simulink model "MODELSIMTOANHETHONG"  (R2020a)
settings: Solver=VariableStepAuto  StartTime=0.0  StopTime=2  RelTol=1e-3
InitFcn:
  | Kp1=65;
  | Ki1=10;
  | Kp2=65;
  | Ki2=45;
  | Kp3=60;
  | Ki3=30;
  | Kp4=60;
  | Ki4=25;
  | Phir=0.2;
undefined symbols (not defined in the file): DiscIntNeverNeededParam, sigbuilder_block
libraries: powerlib x11, modelsimlib x8
settings Model: Creator=Admin  LastModifiedBy=Admin
settings SolverCC: ZeroCrossAlgorithm=Adaptive
settings DebuggingCC: IgnoredZcDiagnostic=none  UnconnectedInputMsg=none  UnconnectedOutputMsg=none  UnconnectedLineMsg=none
settings ModelReferenceCC: EnableRefExpFcnMdlSchedulingChecks=off
settings RTWCC: Description=Generic Real-Time Target

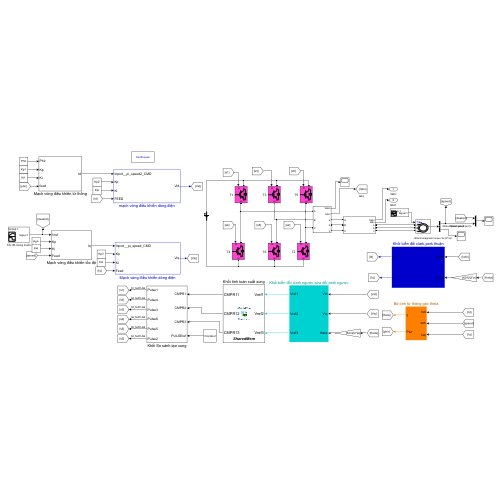
[thumbnail: Simulink's stored preview of the top-level diagram]
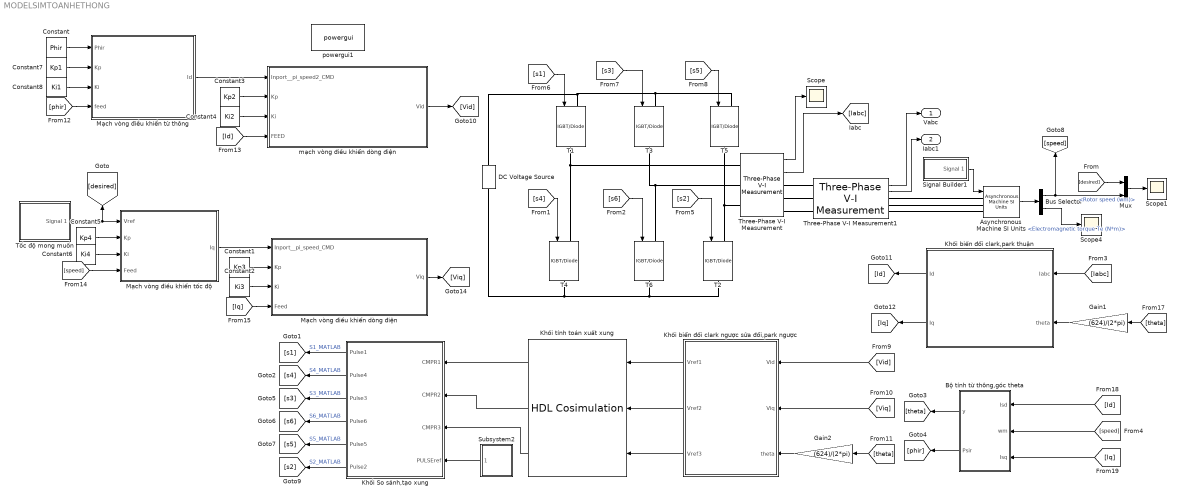
== system MODELSIMTOANHETHONG ==
  Asynchronous Machine SI Units : powerlib/Machines/Asynchronous Machine SI Units  RotorType=Squirrel-cage  PresetModel=No  MechanicalLoad=Torque Tm  ShowDetailedParameters=on  ReferenceFrame=Rotor  Units=SI  MeasurementBus=off  NominalParameters=[40000 380 50]  VoltageRatio=1  Stator=[1.912 0.005974]  Rotor=[1.112 0.005974]  Cage1=[ 0.022 0.226/377]  Cage2=[ 0.022 0.226/377]  Lm=0.2358  Mechanical=[0.4 0 2]  PolePairs=2  InitialConditions=[1 0 0 0 0 0 0 0]  SimulateSaturation=off  Saturation=[14.03593122, 27.81365428, 53.79336849, 72.68890987, 97.98006896, 148.6815601, 215.7428561, 302.9841135, 420.4778367 ; 230, 322, 414, 460, 506, 552, 598, 644, 690]  LoadFlowParameters=1492000  TsPowergui=0  TsBlock=-1  IterativeModel=Trapezoidal non iterative  IterativeDiscreteModel=Trapezoidal non iterative  Pmec=1.492e+006
  Bus Selector : BusSelector  OutputSignals=Mechanical.Rotor speed (wm),Mechanical.Electromagnetic torque Te (N*m)
  Bộ tính từ thông,góc theta : Subsystem
  Constant : Constant  Value=Phir
  Constant1 : Constant  Value=Kp3
  Constant2 : Constant  Value=Ki3
  Constant3 : Constant  Value=Kp2
  Constant4 : Constant  Value=Ki2
  Constant5 : Constant  Value=Kp4
  Constant6 : Constant  Value=Ki4
  Constant7 : Constant  Value=Kp1
  Constant8 : Constant  Value=Ki1
  DC Voltage Source : powerlib/Electrical Sources/DC Voltage Source  Amplitude=515  Measurements=None
  Gain1 : Gain  Gain=(624)/(2*pi)
  Gain2 : Gain  Gain=(624)/(2*pi)
  Khối So sánh,tạo xung : Subsystem
  Khối biến đổi clark,park thuận : Subsystem
  Khối biển đổi clark ngược sửa đổi,park ngược : Subsystem
  Khối tính toán xuất xung : modelsimlib/HDL Cosimulation  PortPaths=/cmpr/Vref1;/cmpr/Vref2;/cmpr/Vref3;/cmpr/CMPR11;/cmpr/CMPR12;/cmpr/CMPR13  PortModes=[1 1 1 2 2 2 ]  PortTimes=[-1,-1,-1,2e-7,2e-7,2e-7]  PortSigns=[-1 -1 -1 -1 -1 -1 ]  PortFracLengths=[0,0,0,0,0,0]  PortWordLengths=[-1,-1,-1,24,24,24]  PortHDLWordSizes=[12,12,12,24,24,24]  CommLocal=on  CommSharedMemory=on  CommPortNumber=4449  CommShowInfo=on  ClockPaths=/cmpr/clk;/cmpr/clk200n  ClockModes=[2 2 ]  ClockTimes=[100e-9,100e-9]  TclPreSimCommand="puts \"Running Simulink Cosimulation block.\""  TclPostSimCommand="puts \"done\""  TimingMode=s  TimingScaleFactor=1  idxCellArray={'UNUSED_VAR'}  CosimBypass=Full Simulation  AllowDirectFeedthrough=on  ProductName=EDA Simulator Link MQ  RunAutoTimescale=off  HdlClocks=0  PreRunTime=0  PreRunTimeUnit=ns
  Mux : Mux  Inputs=2
  Mạch vòng điều khiển dòng điện : Subsystem
  Mạch vòng điều khiển tốc độ : Subsystem
  Mạch vòng điều khiển từ thông : Subsystem
  Scope : Scope
  Scope1 : Scope
  Scope4 : Scope
  Signal Builder1 : Subsystem  Tag=STV Subsys  LoadFcn=sigbuilder_block('load');  StartFcn=sigbuilder_block('start');  StopFcn=sigbuilder_block('stop');  ClipboardFcn=sigbuilder_block('clipboard');  mask(Sigbuilder block){tuvar=[0:10]}
      mask help: Simulink:masks:SigbuilderBlock_MD
      mask init:
      | if ~strcmp(get_param(bdroot(gcbh),'SimulationStatus'),'stopped') tuvar = sigbuilder_block('maskInit'); end
      settings: CopyFcn=sigbuilder_block('copy');  DeleteFcn=sigbuilder_block('delete');  ModelCloseFcn=sigbuilder_block('modelClose');  PreSaveFcn=sigbuilder_block('preSave');  PauseFcn=sigbuilder_block('pause');  ContinueFcn=sigbuilder_block('continue');  NameChangeFcn=sigbuilder_block('namechange');  OpenFcn=sigbuilder_block('open',[437.25 153 550.5 359.25 ]);  CloseFcn=sigbuilder_block('close');
      mask Display: plot(0, 0, 100, 100,[2, 2, 32, 32, 2], [68, 8, 8, 68, 68],[32, 2], [38, 38], [32, 19, 2],[53, 60, 44], [32, 17, 17, 2],[16, 16, 31, 31]);txt = getActiveGroup(gcbh);text(2, 100, txt,'verticalAlignment', 'top');
  Subsystem2 : Subsystem
  T{1..6} (6 alike) : powerlib/Power Electronics/IGBT//Diode  Ron=1e-3  Rs=1e5  Cs=inf  Measurements=off
  Three-Phase V-I Measurement : powerlib/Measurements/Three-Phase V-I Measurement  VoltageMeasurement=phase-to-phase  SetLabelV=off  LabelV=Vabc  Vpu=off  VpuLL=off  CurrentMeasurement=yes  SetLabelI=off  LabelI=Iabc  Ipu=off  Pbase=100e6  Vbase=500e3  OutputType=Complex  PhasorSimulation=off  PSBequivalent=0
  Three-Phase V-I Measurement1 : powerlib/Measurements/Three-Phase V-I Measurement  VoltageMeasurement=phase-to-phase  SetLabelV=off  LabelV=Vabc  Vpu=off  VpuLL=off  CurrentMeasurement=yes  SetLabelI=off  LabelI=Iabc  Ipu=off  Pbase=100e6  Vbase=500e3  OutputType=Complex  PhasorSimulation=off  PSBequivalent=0
  Tốc độ mong muốn : Subsystem  Tag=STV Subsys  LoadFcn=sigbuilder_block('load');  StartFcn=sigbuilder_block('start');  StopFcn=sigbuilder_block('stop');  ClipboardFcn=sigbuilder_block('clipboard');  mask(Sigbuilder block){tuvar=[0:10]}
      mask help: Simulink:masks:SigbuilderBlock_MD
      mask init:
      | if ~strcmp(get_param(bdroot(gcbh),'SimulationStatus'),'stopped') tuvar = sigbuilder_block('maskInit'); end
      settings: CopyFcn=sigbuilder_block('copy');  DeleteFcn=sigbuilder_block('delete');  ModelCloseFcn=sigbuilder_block('modelClose');  PreSaveFcn=sigbuilder_block('preSave');  PauseFcn=sigbuilder_block('pause');  ContinueFcn=sigbuilder_block('continue');  NameChangeFcn=sigbuilder_block('namechange');  OpenFcn=sigbuilder_block('open',[437.25 153 550.5 359.25 ]);  CloseFcn=sigbuilder_block('close');
      mask Display: plot(0, 0, 100, 100,[2, 2, 32, 32, 2], [68, 8, 8, 68, 68],[32, 2], [38, 38], [32, 19, 2],[53, 60, 44], [32, 17, 17, 2],[16, 16, 31, 31]);txt = getActiveGroup(gcbh);text(2, 100, txt,'verticalAlignment', 'top');
  mạch vòng điều khiển dòng điện : Subsystem
  powergui1 : powerlib/powergui  Priority=1  SimulationMode=Continuous  SampleTime=50e-6  frequency=60  Iterations=50  frequencyindice=0  Pbase=100e6  ErrMax=1e-4  UnitsV=kV  UnitsW=MW  buscounter=0  FunctionMessages=off  echomessages=off  EnableUseOfTLC=off  CurrentSourceSwitches=off  DisableSnubberDevices=off  DisableRonSwitches=off  DisableVfSwitches=off  DisplayEquations=off  AutomaticDiscreteSolvers=off  SolverType=Tustin/Backward Euler (TBE)  Interpol=off  ExternalGateDelay=off  methode=off  Ts=100  x0status=blocks  SPID=on  SwTol=0  HookPort=off  NonlinearTolerance=1e-4  nMaxIteration=100  ContinueOnMaxIteration=off  RestoreLinks=warning  ResistiveCurrentMeasurement=off  Frange=[0:2:500]  Ylog=off  Xlog=on  ShowGrid=off  save=off  variable=ZData  structure=0  ZoomFFT=off  StartTime=0.0  cycles=1  DisplayStyle=1  fundamental=60  FreqAxis=off  MaxFrequency=1000  frequencyindicesteady=1  RmsSteady=1  display=off
  Vabc : Outport
  Iabc1 : Outport  Port=2
  wires:
  Bus Selector/1 -> [speed], Mux/2  "<Rotor speed (wm)>"
  Bus Selector/2 -> Scope4/1  "<Electromagnetic torque Te (N*m)>"
  [theta] -> Gain2/1
  Mux/1 -> Scope1/1
  Khối tính toán xuất xung/1 -> Khối So sánh,tạo xung/1(CMPR1)
  Khối tính toán xuất xung/2 -> Khối So sánh,tạo xung/2(CMPR2)
  Khối tính toán xuất xung/3 -> Khối So sánh,tạo xung/3(CMPR3)
  Subsystem2/1(PULSEref) -> Khối So sánh,tạo xung/4(PULSEref)
  Khối So sánh,tạo xung/1(Pulse1) -> [s1]  "S1_MATLAB"
  Khối So sánh,tạo xung/2(Pulse4) -> [s4]  "S4_MATLAB"
  Khối So sánh,tạo xung/3(Pulse3) -> [s3]  "S3_MATLAB"
  Khối So sánh,tạo xung/4(Pulse6) -> [s6]  "S6_MATLAB"
  Khối So sánh,tạo xung/5(Pulse5) -> [s5]  "S5_MATLAB"
  Khối So sánh,tạo xung/6(Pulse2) -> [s2]  "S2_MATLAB"
  Three-Phase V-I Measurement/1 -> Scope/1
  [desired] -> Mux/1
  Three-Phase V-I Measurement1/2 -> Iabc1/1
  [s1] -> T1/1
  [s6] -> T6/1
  Three-Phase V-I Measurement1/1 -> Vabc/1
  [s4] -> T4/1
  [s5] -> T5/1
  [s2] -> T2/1
  [s3] -> T3/1
  Signal Builder1/1(Signal 1) -> Asynchronous Machine SI Units/1
  Three-Phase V-I Measurement/2 -> [Iabc]
  Asynchronous Machine SI Units/1 -> Bus Selector/1
  Tốc độ mong muốn/1(Signal 1) -> [desired], Mạch vòng điều khiển tốc độ/1(Vref)
  [Id] -> Bộ tính từ thông,góc theta/1(Isd)
  [speed] -> Bộ tính từ thông,góc theta/2(wm)
  [Iq] -> Bộ tính từ thông,góc theta/3(Isq)
  Bộ tính từ thông,góc theta/1(y) -> [theta]
  Bộ tính từ thông,góc theta/2(Psir) -> [phir]
  [Vid] -> Khối biển đổi clark ngược sửa đổi,park ngược/1(Vid)
  [Viq] -> Khối biển đổi clark ngược sửa đổi,park ngược/2(Viq)
  Gain2/1 -> Khối biển đổi clark ngược sửa đổi,park ngược/3(theta)
  Khối biển đổi clark ngược sửa đổi,park ngược/1(Vref1) -> Khối tính toán xuất xung/1
  Khối biển đổi clark ngược sửa đổi,park ngược/2(Vref2) -> Khối tính toán xuất xung/2
  Khối biển đổi clark ngược sửa đổi,park ngược/3(Vref3) -> Khối tính toán xuất xung/3
  Constant/1 -> Mạch vòng điều khiển từ thông/1(Phir)
  Constant7/1 -> Mạch vòng điều khiển từ thông/2(Kp)
  Constant8/1 -> Mạch vòng điều khiển từ thông/3(Ki)
  [phir] -> Mạch vòng điều khiển từ thông/4(feed)
  Mạch vòng điều khiển từ thông/1(Id) -> mạch vòng điều khiển dòng điện/1(Inport__pi_speed2_CMD)
  Constant3/1 -> mạch vòng điều khiển dòng điện/2(Kp)
  Constant4/1 -> mạch vòng điều khiển dòng điện/3(Ki)
  [Id] -> mạch vòng điều khiển dòng điện/4(FEED)
  mạch vòng điều khiển dòng điện/1(Vid) -> [Vid]
  Constant1/1 -> Mạch vòng điều khiển dòng điện/2(Kp)
  Constant2/1 -> Mạch vòng điều khiển dòng điện/3(Ki)
  [Iq] -> Mạch vòng điều khiển dòng điện/4(Feed)
  Mạch vòng điều khiển dòng điện/1(Viq) -> [Viq]
  Constant5/1 -> Mạch vòng điều khiển tốc độ/2(Kp)
  Constant6/1 -> Mạch vòng điều khiển tốc độ/3(Ki)
  [speed] -> Mạch vòng điều khiển tốc độ/4(Feed)
  Mạch vòng điều khiển tốc độ/1(Iq) -> Mạch vòng điều khiển dòng điện/1(Inport__pi_speed_CMD)
  [theta] -> Gain1/1
  [Iabc] -> Khối biến đổi clark,park thuận/1(Iabc)
  Gain1/1 -> Khối biến đổi clark,park thuận/2(theta)
  Khối biến đổi clark,park thuận/1(Id) -> [Id]
  Khối biến đổi clark,park thuận/2(Iq) -> [Iq]
  connections:
  T2/LConn1 -- Three-Phase V-I Measurement/LConn3 -- T5/RConn1
  T6/LConn1 -- T3/RConn1 -- Three-Phase V-I Measurement/LConn2
  T1/LConn1 -- T5/LConn1 -- T3/LConn1 -- DC Voltage Source/RConn1
  T2/RConn1 -- DC Voltage Source/LConn1 -- T4/RConn1 -- T6/RConn1
  T4/LConn1 -- Three-Phase V-I Measurement/LConn1 -- T1/RConn1
  Three-Phase V-I Measurement/RConn3 -- Three-Phase V-I Measurement1/LConn3
  Asynchronous Machine SI Units/LConn2 -- Three-Phase V-I Measurement1/RConn2
  Asynchronous Machine SI Units/LConn1 -- Three-Phase V-I Measurement1/RConn1
  Asynchronous Machine SI Units/LConn3 -- Three-Phase V-I Measurement1/RConn3
  Three-Phase V-I Measurement/RConn1 -- Three-Phase V-I Measurement1/LConn1
  Three-Phase V-I Measurement1/LConn2 -- Three-Phase V-I Measurement/RConn2

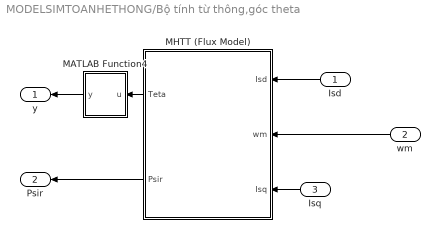
== system MODELSIMTOANHETHONG/Bộ tính từ thông,góc theta ==
  Isd : Inport
  wm : Inport  Port=2
  Isq : Inport  Port=3
  MATLAB Function4 : MATLAB Function  TreatAsAtomicUnit=on
  MHTT (Flux Model) : Subsystem
  y : Outport
  Psir : Outport  Port=2
  wires:
  wm/1 -> MHTT (Flux Model)/2(wm)
  MHTT (Flux Model)/1(Teta) -> MATLAB Function4/1(u)
  Isq/1 -> MHTT (Flux Model)/3(Isq)
  Isd/1 -> MHTT (Flux Model)/1(Isd)
  MATLAB Function4/1(y) -> y/1
  MHTT (Flux Model)/2(Psir) -> Psir/1

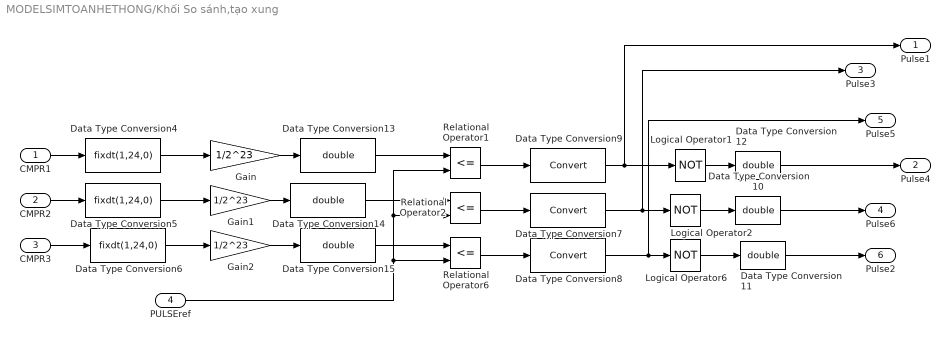
== system MODELSIMTOANHETHONG/Khối So sánh,tạo xung ==
  CMPR1 : Inport
  CMPR2 : Inport  Port=2
  CMPR3 : Inport  Port=3
  PULSEref : Inport  Port=4
  Data Type Conversion10 : DataTypeConversion  OutDataTypeStr=double
  Data Type Conversion11 : DataTypeConversion  OutDataTypeStr=double
  Data Type Conversion12 : DataTypeConversion  OutDataTypeStr=double
  Data Type Conversion13 : DataTypeConversion  OutDataTypeStr=double  SampleTime=2e-7
  Data Type Conversion14 : DataTypeConversion  OutDataTypeStr=double  SampleTime=2e-7
  Data Type Conversion15 : DataTypeConversion  OutDataTypeStr=double  SampleTime=2e-7
  Data Type Conversion4 : DataTypeConversion  OutDataTypeStr=fixdt(1,24,0)  SampleTime=2e-7
  Data Type Conversion5 : DataTypeConversion  OutDataTypeStr=fixdt(1,24,0)  SampleTime=2e-7
  Data Type Conversion6 : DataTypeConversion  OutDataTypeStr=fixdt(1,24,0)  SampleTime=2e-7
  Data Type Conversion7 : DataTypeConversion
  Data Type Conversion8 : DataTypeConversion
  Data Type Conversion9 : DataTypeConversion
  Gain : Gain  Gain=1/2^23
  Gain1 : Gain  Gain=1/2^23
  Gain2 : Gain  Gain=1/2^23
  Logical Operator1 : Logic  Operator=NOT  AllPortsSameDT=off
  Logical Operator2 : Logic  Operator=NOT  AllPortsSameDT=off
  Logical Operator6 : Logic  Operator=NOT  AllPortsSameDT=off
  Relational Operator1 : RelationalOperator  Operator=<=  OutDataTypeStr=boolean  RndMeth=Simplest
  Relational Operator2 : RelationalOperator  Operator=<=  OutDataTypeStr=boolean  RndMeth=Simplest
  Relational Operator6 : RelationalOperator  Operator=<=  OutDataTypeStr=boolean  RndMeth=Simplest
  Pulse1 : Outport
  Pulse4 : Outport  Port=2
  Pulse3 : Outport  Port=3
  Pulse6 : Outport  Port=4
  Pulse5 : Outport  Port=5
  Pulse2 : Outport  Port=6
  wires:
  Logical Operator2/1 -> Data Type Conversion10/1
  Logical Operator6/1 -> Data Type Conversion11/1
  PULSEref/1 -> Relational Operator6/2, Relational Operator2/2, Relational Operator1/2
  Relational Operator1/1 -> Data Type Conversion9/1
  Data Type Conversion9/1 -> Pulse1/1, Logical Operator1/1
  Relational Operator6/1 -> Data Type Conversion8/1
  Relational Operator2/1 -> Data Type Conversion7/1
  Data Type Conversion8/1 -> Pulse5/1, Logical Operator6/1
  Logical Operator1/1 -> Data Type Conversion12/1
  Data Type Conversion7/1 -> Pulse3/1, Logical Operator2/1
  Data Type Conversion12/1 -> Pulse4/1
  Data Type Conversion10/1 -> Pulse6/1
  Data Type Conversion11/1 -> Pulse2/1
  Gain1/1 -> Data Type Conversion14/1
  Data Type Conversion5/1 -> Gain1/1
  Gain2/1 -> Data Type Conversion15/1
  Data Type Conversion4/1 -> Gain/1
  Data Type Conversion6/1 -> Gain2/1
  Gain/1 -> Data Type Conversion13/1
  Data Type Conversion13/1 -> Relational Operator1/1
  CMPR1/1 -> Data Type Conversion4/1
  CMPR2/1 -> Data Type Conversion5/1
  Data Type Conversion14/1 -> Relational Operator2/1
  CMPR3/1 -> Data Type Conversion6/1
  Data Type Conversion15/1 -> Relational Operator6/1

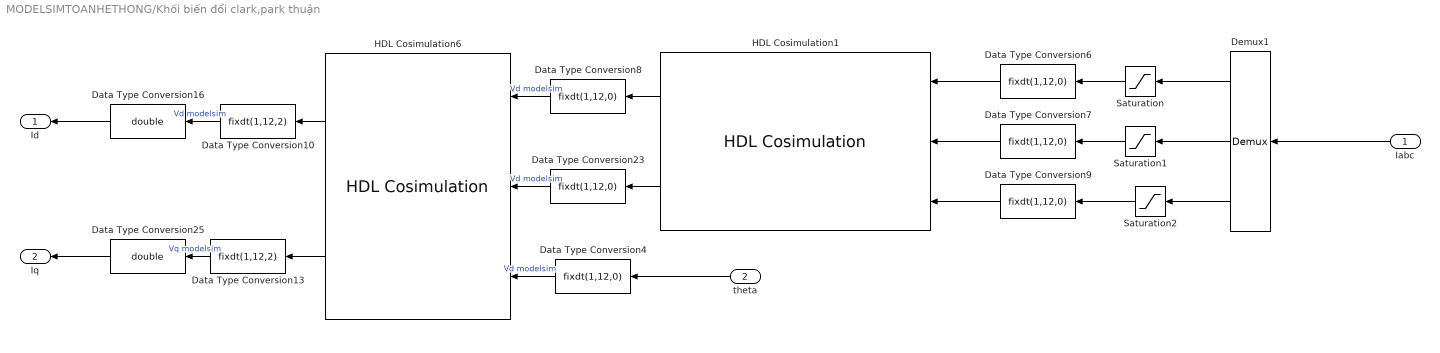
== system MODELSIMTOANHETHONG/Khối biến đổi clark,park thuận ==
  Iabc : Inport
  theta : Inport  Port=2
  Data Type Conversion10 : DataTypeConversion  OutDataTypeStr=fixdt(1,12,2)  SampleTime=2e-7
  Data Type Conversion13 : DataTypeConversion  OutDataTypeStr=fixdt(1,12,2)  SampleTime=2e-7
  Data Type Conversion16 : DataTypeConversion  OutDataTypeStr=double  SampleTime=2e-7
  Data Type Conversion{4,6..9,23} (6 alike) : DataTypeConversion  OutDataTypeStr=fixdt(1,12,0)  SampleTime=2e-7
  Data Type Conversion25 : DataTypeConversion  OutDataTypeStr=double  SampleTime=2e-7
  Demux1 : Demux  Outputs=3
  HDL Cosimulation1 : modelsimlib/HDL Cosimulation  PortPaths=/clark/V1;/clark/V2;/clark/V3;/clark/Va;/clark/Vb  PortModes=[1 1 1 2 2 ]  PortTimes=[-1,-1,-1,2e-7,2e-7]  PortSigns=[-1 -1 -1 -1 -1 ]  PortFracLengths=[0,0,0,0,0]  PortWordLengths=[-1,-1,-1,12,12]  PortHDLWordSizes=[12,12,12,12,12]  CommLocal=on  CommSharedMemory=on  CommPortNumber=4449  CommShowInfo=on  ClockPaths=/clark/clk;/clark/clk80n  ClockModes=[2 2 ]  ClockTimes=[100e-9,100e-9]  TclPreSimCommand="puts \"Running Simulink Cosimulation block.\""  TclPostSimCommand="puts \"done\""  TimingMode=s  TimingScaleFactor=1  idxCellArray={'UNUSED_VAR'}  CosimBypass=Full Simulation  AllowDirectFeedthrough=on  ProductName=EDA Simulator Link MQ  RunAutoTimescale=off  HdlClocks=0  PreRunTime=0  PreRunTimeUnit=ns
  HDL Cosimulation6 : modelsimlib/HDL Cosimulation  PortPaths=/park/Va;/park/Vb;/park/ADDRESS;/park/Vd;/park/Vq  PortModes=[1 1 1 2 2 ]  PortTimes=[-1,-1,-1,2e-7,2e-7]  PortSigns=[-1 -1 -1 -1 -1 ]  PortFracLengths=[0,0,0,0,0]  PortWordLengths=[-1,-1,-1,12,12]  PortHDLWordSizes=[12,12,12,12,12]  CommLocal=on  CommSharedMemory=on  CommPortNumber=4449  CommShowInfo=on  ClockPaths=/park/clk;/park/clk80n  ClockModes=[2 2 ]  ClockTimes=[100e-9,100e-9]  TclPreSimCommand="puts \"Running Simulink Cosimulation block.\""  TclPostSimCommand="puts \"done\""  TimingMode=s  TimingScaleFactor=1  idxCellArray={'UNUSED_VAR'}  CosimBypass=Full Simulation  AllowDirectFeedthrough=on  ProductName=EDA Simulator Link MQ  RunAutoTimescale=off  HdlClocks=0  PreRunTime=0  PreRunTimeUnit=ns
  Saturation : Saturate  UpperLimit=2048  LowerLimit=-2047
  Saturation1 : Saturate  UpperLimit=2048  LowerLimit=-2047
  Saturation2 : Saturate  UpperLimit=2048  LowerLimit=-2047
  Id : Outport
  Iq : Outport  Port=2
  wires:
  Data Type Conversion9/1 -> HDL Cosimulation1/3
  HDL Cosimulation6/2 -> Data Type Conversion13/1
  HDL Cosimulation1/2 -> Data Type Conversion23/1
  Data Type Conversion7/1 -> HDL Cosimulation1/2
  Saturation2/1 -> Data Type Conversion9/1
  Saturation/1 -> Data Type Conversion6/1
  Data Type Conversion6/1 -> HDL Cosimulation1/1
  Data Type Conversion8/1 -> HDL Cosimulation6/1  "Vd modelsim"
  Data Type Conversion4/1 -> HDL Cosimulation6/3  "Vd modelsim"
  Demux1/2 -> Saturation1/1
  theta/1 -> Data Type Conversion4/1
  HDL Cosimulation1/1 -> Data Type Conversion8/1
  Data Type Conversion13/1 -> Data Type Conversion25/1  "Vq modelsim"
  Demux1/1 -> Saturation/1
  Saturation1/1 -> Data Type Conversion7/1
  Data Type Conversion10/1 -> Data Type Conversion16/1  "Vd modelsim"
  HDL Cosimulation6/1 -> Data Type Conversion10/1
  Demux1/3 -> Saturation2/1
  Data Type Conversion25/1 -> Iq/1
  Data Type Conversion23/1 -> HDL Cosimulation6/2  "Vd modelsim"
  Data Type Conversion16/1 -> Id/1
  Iabc/1 -> Demux1/1

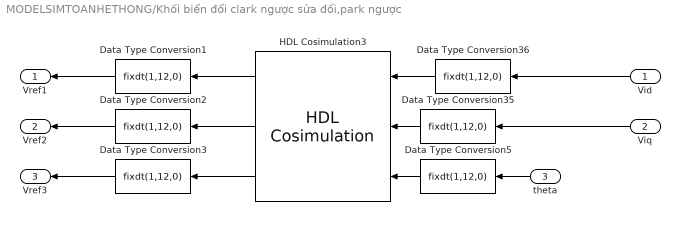
== system MODELSIMTOANHETHONG/Khối biển đổi clark ngược sửa đổi,park ngược ==
  Vid : Inport
  Viq : Inport  Port=2
  theta : Inport  Port=3
  Data Type Conversion{1..3,5,35..36} (6 alike) : DataTypeConversion  OutDataTypeStr=fixdt(1,12,0)  SampleTime=2e-7
  HDL Cosimulation3 : modelsimlib/HDL Cosimulation  PortPaths=/sin_cos/CMD_ID;/sin_cos/CMD_IQ;/sin_cos/ADDRESS;/sin_cos/Vref1;/sin_cos/Vref2;/sin_cos/Vref3  PortModes=[1 1 1 2 2 2 ]  PortTimes=[-1,-1,-1,2e-7,2e-7,2e-7]  PortSigns=[-1 -1 -1 -1 -1 -1 ]  PortFracLengths=[0,0,0,0,0,0]  PortWordLengths=[-1,-1,-1,12,12,12]  PortHDLWordSizes=[12,12,12,12,12,12]  CommLocal=on  CommSharedMemory=on  CommPortNumber=4449  CommShowInfo=on  ClockPaths=/sin_cos/clk;/sin_cos/clk80n  ClockModes=[2 2 ]  ClockTimes=[100e-9,100e-9]  TclPreSimCommand="puts \"Running Simulink Cosimulation block.\""  TclPostSimCommand="puts \"done\""  TimingMode=s  TimingScaleFactor=1  idxCellArray={'UNUSED_VAR'}  CosimBypass=Full Simulation  AllowDirectFeedthrough=on  ProductName=EDA Simulator Link MQ  RunAutoTimescale=off  HdlClocks=0  PreRunTime=0  PreRunTimeUnit=ns
  Vref1 : Outport
  Vref2 : Outport  Port=2
  Vref3 : Outport  Port=3
  wires:
  Data Type Conversion3/1 -> Vref3/1
  HDL Cosimulation3/2 -> Data Type Conversion2/1
  Data Type Conversion5/1 -> HDL Cosimulation3/3
  HDL Cosimulation3/1 -> Data Type Conversion1/1
  Data Type Conversion35/1 -> HDL Cosimulation3/2
  Data Type Conversion1/1 -> Vref1/1
  Viq/1 -> Data Type Conversion35/1
  HDL Cosimulation3/3 -> Data Type Conversion3/1
  Data Type Conversion36/1 -> HDL Cosimulation3/1
  Data Type Conversion2/1 -> Vref2/1
  Vid/1 -> Data Type Conversion36/1
  theta/1 -> Data Type Conversion5/1

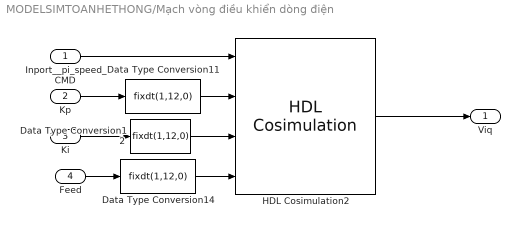
== system MODELSIMTOANHETHONG/Mạch vòng điều khiển dòng điện ==
  Inport__pi_speed_CMD : Inport
  Kp : Inport  Port=2
  Ki : Inport  Port=3
  Feed : Inport  Port=4
  Data Type Conversion11 : DataTypeConversion  OutDataTypeStr=fixdt(1,12,0)  SampleTime=2e-7
  Data Type Conversion12 : DataTypeConversion  OutDataTypeStr=fixdt(1,12,0)  SampleTime=2e-7
  Data Type Conversion14 : DataTypeConversion  OutDataTypeStr=fixdt(1,12,0)  SampleTime=2e-7
  HDL Cosimulation2 : modelsimlib/HDL Cosimulation  PortPaths=/pi_speed/CMD;/pi_speed/Kp;/pi_speed/Ki;/pi_speed/Feed;/pi_speed/daura  PortModes=[1 1 1 1 2 ]  PortTimes=[-1,-1,-1,-1,2e-7]  PortSigns=[-1 -1 -1 -1 -1 ]  PortFracLengths=[0,0,0,0,0]  PortWordLengths=[-1,-1,-1,-1,12]  PortHDLWordSizes=[12,12,12,12,12]  CommLocal=on  CommSharedMemory=on  CommPortNumber=4449  CommShowInfo=on  ClockPaths=/pi_speed/clk;/pi_speed/clk40  ClockModes=[2 2 ]  ClockTimes=[100e-9,100e-9]  TclPreSimCommand="puts \"Running Simulink Cosimulation block.\""  TclPostSimCommand="puts \"done\""  TimingMode=s  TimingScaleFactor=1  idxCellArray={'UNUSED_VAR'}  CosimBypass=Full Simulation  AllowDirectFeedthrough=on  ProductName=EDA Simulator Link MQ  RunAutoTimescale=off  HdlClocks=0  PreRunTime=0  PreRunTimeUnit=ns
  Viq : Outport
  wires:
  Data Type Conversion14/1 -> HDL Cosimulation2/4
  Data Type Conversion12/1 -> HDL Cosimulation2/3
  HDL Cosimulation2/1 -> Viq/1
  Data Type Conversion11/1 -> HDL Cosimulation2/2
  Ki/1 -> Data Type Conversion12/1
  Feed/1 -> Data Type Conversion14/1
  Inport__pi_speed_CMD/1 -> HDL Cosimulation2/1
  Kp/1 -> Data Type Conversion11/1

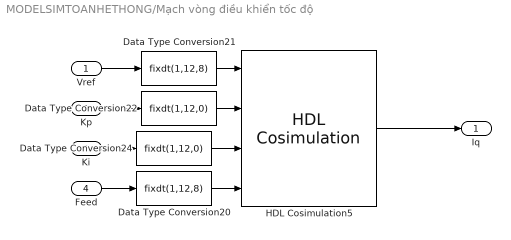
== system MODELSIMTOANHETHONG/Mạch vòng điều khiển tốc độ ==
  Vref : Inport
  Kp : Inport  Port=2
  Ki : Inport  Port=3
  Feed : Inport  Port=4
  Data Type Conversion20 : DataTypeConversion  OutDataTypeStr=fixdt(1,12,8)  SampleTime=2e-7
  Data Type Conversion21 : DataTypeConversion  OutDataTypeStr=fixdt(1,12,8)  SampleTime=2e-7
  Data Type Conversion22 : DataTypeConversion  OutDataTypeStr=fixdt(1,12,0)  SampleTime=2e-7
  Data Type Conversion24 : DataTypeConversion  OutDataTypeStr=fixdt(1,12,0)  SampleTime=2e-7
  HDL Cosimulation5 : modelsimlib/HDL Cosimulation  PortPaths=/pi_speed1/CMD;/pi_speed1/Kp;/pi_speed1/Ki;/pi_speed1/Feed;/pi_speed1/daura  PortModes=[1 1 1 1 2 ]  PortTimes=[-1,-1,-1,-1,2e-7]  PortSigns=[-1 -1 -1 -1 -1 ]  PortFracLengths=[0,0,0,0,0]  PortWordLengths=[-1,-1,-1,-1,12]  PortHDLWordSizes=[12,12,12,12,12]  CommLocal=on  CommSharedMemory=on  CommPortNumber=4449  CommShowInfo=on  ClockPaths=/pi_speed1/clk;/pi_speed1/clk40  ClockModes=[2 2 ]  ClockTimes=[100e-9,100e-9]  TclPreSimCommand="puts \"Running Simulink Cosimulation block.\""  TclPostSimCommand="puts \"done\""  TimingMode=s  TimingScaleFactor=1  idxCellArray={'UNUSED_VAR'}  CosimBypass=Full Simulation  AllowDirectFeedthrough=on  ProductName=EDA Simulator Link MQ  RunAutoTimescale=off  HdlClocks=0  PreRunTime=0  PreRunTimeUnit=ns
  Iq : Outport
  wires:
  Feed/1 -> Data Type Conversion20/1
  Data Type Conversion22/1 -> HDL Cosimulation5/2
  Ki/1 -> Data Type Conversion24/1
  Data Type Conversion21/1 -> HDL Cosimulation5/1
  Vref/1 -> Data Type Conversion21/1
  Data Type Conversion20/1 -> HDL Cosimulation5/4
  HDL Cosimulation5/1 -> Iq/1
  Data Type Conversion24/1 -> HDL Cosimulation5/3
  Kp/1 -> Data Type Conversion22/1

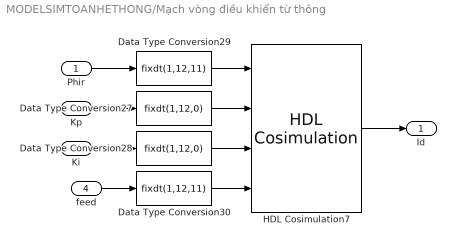
== system MODELSIMTOANHETHONG/Mạch vòng điều khiển từ thông ==
  Phir : Inport
  Kp : Inport  Port=2
  Ki : Inport  Port=3
  feed : Inport  Port=4
  Data Type Conversion27 : DataTypeConversion  OutDataTypeStr=fixdt(1,12,0)  SampleTime=2e-7
  Data Type Conversion28 : DataTypeConversion  OutDataTypeStr=fixdt(1,12,0)  SampleTime=2e-7
  Data Type Conversion29 : DataTypeConversion  OutDataTypeStr=fixdt(1,12,11)  SampleTime=2e-7
  Data Type Conversion30 : DataTypeConversion  OutDataTypeStr=fixdt(1,12,11)  SampleTime=2e-7
  HDL Cosimulation7 : modelsimlib/HDL Cosimulation  PortPaths=/pi_speed4/CMD;/pi_speed4/Kp;/pi_speed4/Ki;/pi_speed4/FEED;/pi_speed4/DAURA  PortModes=[1 1 1 1 2 ]  PortTimes=[-1,-1,-1,-1,2e-7]  PortSigns=[-1 -1 -1 -1 -1 ]  PortFracLengths=[0,0,0,0,0]  PortWordLengths=[-1,-1,-1,-1,12]  PortHDLWordSizes=[12,12,12,12,12]  CommLocal=on  CommSharedMemory=on  CommPortNumber=4449  CommShowInfo=on  ClockPaths=/pi_speed4/clk;/pi_speed4/clk40  ClockModes=[2 2 ]  ClockTimes=[100e-9,100e-9]  TclPreSimCommand="puts \"Running Simulink Cosimulation block.\""  TclPostSimCommand="puts \"done\""  TimingMode=s  TimingScaleFactor=1  idxCellArray={'UNUSED_VAR'}  CosimBypass=Full Simulation  AllowDirectFeedthrough=on  ProductName=EDA Simulator Link MQ  RunAutoTimescale=off  HdlClocks=0  PreRunTime=0  PreRunTimeUnit=ns
  Id : Outport
  wires:
  Data Type Conversion30/1 -> HDL Cosimulation7/4
  Phir/1 -> Data Type Conversion29/1
  HDL Cosimulation7/1 -> Id/1
  Data Type Conversion29/1 -> HDL Cosimulation7/1
  Kp/1 -> Data Type Conversion27/1
  Data Type Conversion28/1 -> HDL Cosimulation7/3
  Data Type Conversion27/1 -> HDL Cosimulation7/2
  Ki/1 -> Data Type Conversion28/1
  feed/1 -> Data Type Conversion30/1

== system MODELSIMTOANHETHONG/Signal Builder1 ==
  Demux : Demux  Tag=STV Demux  Outputs=1
      settings: DisplayOption=none
  FromWs : FromWorkspace  Tag=STV FromWs  VariableName=tuvar
      SigBuilderData=|
      | common.afterFinalStr = 'Extrapolate'
      | common.sampleTime = 0
      | dataSet.timeRange = [0 10]
      | dataSet.name = 'Group 1'
      | sbobj.Groups.Name = 'Group 1'
      | sbobj.Groups.Signals.Name = 'Signal 1'
      | sbobj.Groups.Signals.XData = [0 2 2 2.5 2.5 10]
      | sbobj.Groups.Signals.YData = [0 0 5 5 0 0]
  Signal 1 : Outport  Tag=STV Outport  VectorParamsAs1DForOutWhenUnconnected=off
  wires:
  Demux/1 -> Signal 1/1
  FromWs/1 -> Demux/1

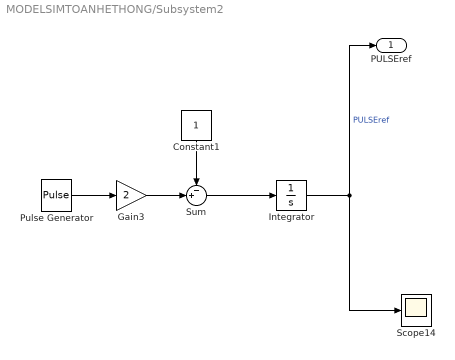
== system MODELSIMTOANHETHONG/Subsystem2 ==
  Constant1 : Constant
  Gain3 : Gain  Gain=2
  Integrator : Integrator
  Pulse Generator : DiscretePulseGenerator  PulseType=Time based  Period=1e-4 * 2  PulseWidth=50
  Scope14 : Scope
  Sum : Sum  Inputs=-+|
  PULSEref : Outport
  wires:
  Pulse Generator/1 -> Gain3/1
  Constant1/1 -> Sum/1
  Integrator/1 -> PULSEref/1, Scope14/1  "PULSEref"
  Sum/1 -> Integrator/1
  Gain3/1 -> Sum/2

== system MODELSIMTOANHETHONG/Tốc độ mong muốn ==
  Demux : Demux  Tag=STV Demux  Outputs=1
      settings: DisplayOption=none
  FromWs : FromWorkspace  Tag=STV FromWs  VariableName=tuvar
      SigBuilderData=|
      | common.afterFinalStr = 'Extrapolate'
      | common.sampleTime = 0
      | dataSet.timeRange = [0 2]
      | dataSet.name = 'Group 1'
      | sbobj.Groups.Name = 'Group 1'
      | sbobj.Groups.Signals.Name = 'Signal 1'
      | sbobj.Groups.Signals.XData = [0 0.5 0.9 1.4 1.8 2]
      | sbobj.Groups.Signals.YData = [0 5 5 -5 -5 0]
      | sbobj.Groups.TimeRange = [0 2]
  Signal 1 : Outport  Tag=STV Outport  VectorParamsAs1DForOutWhenUnconnected=off
  wires:
  Demux/1 -> Signal 1/1
  FromWs/1 -> Demux/1

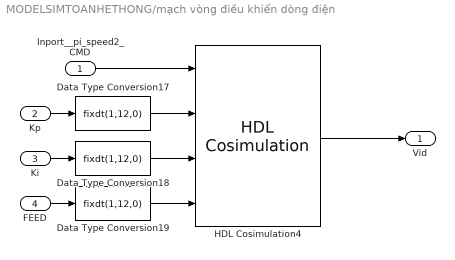
== system MODELSIMTOANHETHONG/mạch vòng điều khiển dòng điện ==
  Inport__pi_speed2_CMD : Inport
  Kp : Inport  Port=2
  Ki : Inport  Port=3
  FEED : Inport  Port=4
  Data Type Conversion17 : DataTypeConversion  OutDataTypeStr=fixdt(1,12,0)  SampleTime=2e-7
  Data Type Conversion18 : DataTypeConversion  OutDataTypeStr=fixdt(1,12,0)  SampleTime=2e-7
  Data Type Conversion19 : DataTypeConversion  OutDataTypeStr=fixdt(1,12,0)  SampleTime=2e-7
  HDL Cosimulation4 : modelsimlib/HDL Cosimulation  PortPaths=/pi_speed2/CMD;/pi_speed2/Kp;/pi_speed2/Ki;/pi_speed2/FEED;/pi_speed2/DAURA  PortModes=[1 1 1 1 2 ]  PortTimes=[-1,-1,-1,-1,2e-7]  PortSigns=[-1 -1 -1 -1 -1 ]  PortFracLengths=[0,0,0,0,0]  PortWordLengths=[-1,-1,-1,-1,-1]  PortHDLWordSizes=[0,0,0,0,0]  CommLocal=on  CommSharedMemory=on  CommPortNumber=4449  CommShowInfo=on  ClockPaths=/pi_speed2/clk;/pi_speed2/clk40  ClockModes=[2 2 ]  ClockTimes=[100e-9,100e-9]  TclPreSimCommand="puts \"Running Simulink Cosimulation block.\""  TclPostSimCommand="puts \"done\""  TimingMode=s  TimingScaleFactor=1  idxCellArray={'UNUSED_VAR'}  CosimBypass=Full Simulation  AllowDirectFeedthrough=on  ProductName=EDA Simulator Link MQ  RunAutoTimescale=off  HdlClocks=0  PreRunTime=0  PreRunTimeUnit=ns
  Vid : Outport
  wires:
  Kp/1 -> Data Type Conversion17/1
  HDL Cosimulation4/1 -> Vid/1
  Data Type Conversion19/1 -> HDL Cosimulation4/4
  FEED/1 -> Data Type Conversion19/1
  Inport__pi_speed2_CMD/1 -> HDL Cosimulation4/1
  Data Type Conversion17/1 -> HDL Cosimulation4/2
  Data Type Conversion18/1 -> HDL Cosimulation4/3
  Ki/1 -> Data Type Conversion18/1

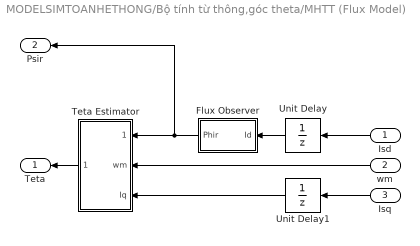
== system MODELSIMTOANHETHONG/Bộ tính từ thông,góc theta/MHTT (Flux Model) ==
  Isd : Inport
  wm : Inport  Port=2
  Isq : Inport  Port=3
  Flux Observer : Subsystem  mask(Flux Calcultation){}
      mask init:
      | NF=0.44572610323020e-6;
      | DF=[1 -0.99998715486734];
  Teta Estimator : Subsystem
  Unit Delay : UnitDelay  SampleTime=-1  HasFrameUpgradeWarning=on
  Unit Delay1 : UnitDelay  SampleTime=-1  HasFrameUpgradeWarning=on
  Teta : Outport  VectorParamsAs1DForOutWhenUnconnected=off
  Psir : Outport  Port=2  VectorParamsAs1DForOutWhenUnconnected=off
  wires:
  Unit Delay1/1 -> Teta Estimator/3(Iq)
  Teta Estimator/1(Teta) -> Teta/1
  wm/1 -> Teta Estimator/2(wm)
  Isd/1 -> Unit Delay/1
  Unit Delay/1 -> Flux Observer/1(Id)
  Flux Observer/1(Phir) -> Psir/1, Teta Estimator/1(Phird)
  Isq/1 -> Unit Delay1/1

== system MODELSIMTOANHETHONG/Bộ tính từ thông,góc theta/MHTT (Flux Model)/Flux Observer ==
  note: Phir = Lm *Id / (1 +Tr .s)
  note: Lm = 34.7 mH
  note: Lr = Ll'r +Lm = 0.8 +34.7= 35.5 mH
  note: Tr = Lr / Rr = 0.1557 s
  note: Rr = 0.228 ohms
  Id : Inport
  Discrete Tranfer Function : Subsystem  mask(First Order Low Pass Filter (Discrete)){T=0.1557, Ts=0.001}
      mask prompts: T "Time constant T (s) :"; Ts "Time step (s)"
      mask help: H(s)=1/(1+T.s)
      mask init:
      | X=[0 1 2 3 4];
      |  Y=[-2 -2 -3 -4 -4];
      |  str=sprintf('\nH=1/(1+T.s)\n T= %g s\n\n\n',T);
      | num=1;
      | den=[T 1];
      | 
      | % discrete transfer function
      | % descending powers of z
      | numd= Ts/T;
      | dend=[ 1  (Ts-T)/T];
      mask Display:
      | plot(X,Y);
      | disp(str);
  Lm : Gain  Gain=34.7e-3  SaturateOnIntegerOverflow=on  OutDataTypeStr=Inherit: Same as input  ParamDataTypeStr=Inherit: Same as input
  Phir : Outport  VectorParamsAs1DForOutWhenUnconnected=off
  wires:
  Discrete Tranfer Function/1(Out) -> Phir/1
  Id/1 -> Lm/1
  Lm/1 -> Discrete Tranfer Function/1(In)

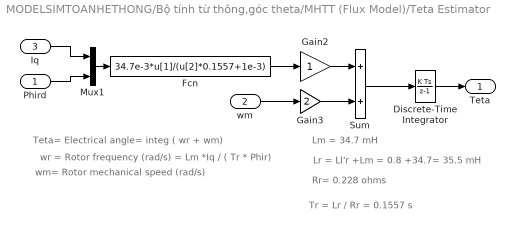
== system MODELSIMTOANHETHONG/Bộ tính từ thông,góc theta/MHTT (Flux Model)/Teta Estimator ==
  note: Teta= Electrical angle= integ ( wr + wm)
  note: wr = Rotor frequency (rad/s) = Lm *Iq / ( Tr * Phir)
  note: Lm = 34.7 mH
  note: Rr= 0.228 ohms
  note: Lr = Ll'r +Lm = 0.8 +34.7= 35.5 mH
  note: wm= Rotor mechanical speed (rad/s)
  note: Tr = Lr / Rr = 0.1557 s
  Phird : Inport
  wm : Inport  Port=2
  Iq : Inport  Port=3
  Discrete-Time Integrator : DiscreteIntegrator  SampleTime=-1  ICPrevOutput=DiscIntNeverNeededParam  ICPrevScaledInput=DiscIntNeverNeededParam
  Fcn : Fcn  Expr=34.7e-3*u[1]/(u[2]*0.1557+1e-3)
  Gain2 : Gain  SaturateOnIntegerOverflow=on  OutDataTypeStr=Inherit: Same as input  ParamDataTypeStr=Inherit: Same as input
  Gain3 : Gain  Gain=2  SaturateOnIntegerOverflow=on  OutDataTypeStr=Inherit: Same as input  ParamDataTypeStr=Inherit: Same as input
  Mux1 : Mux  Inputs=2
  Sum : Sum  InputSameDT=on  SaturateOnIntegerOverflow=on  OutDataTypeStr=Inherit: Same as first input
  Teta : Outport  InitialOutput=0  VectorParamsAs1DForOutWhenUnconnected=off
  wires:
  Discrete-Time Integrator/1 -> Teta/1
  Sum/1 -> Discrete-Time Integrator/1
  Gain3/1 -> Sum/2
  Gain2/1 -> Sum/1
  wm/1 -> Gain3/1
  Fcn/1 -> Gain2/1
  Phird/1 -> Mux1/2
  Iq/1 -> Mux1/1
  Mux1/1 -> Fcn/1

== system MODELSIMTOANHETHONG/Bộ tính từ thông,góc theta/MHTT (Flux Model)/Flux Observer/Discrete Tranfer Function ==
  In : Inport
  Discrete Transfer Fcn : DiscreteTransferFcn  Numerator=numd  Denominator=dend  SampleTime=Ts
  Out : Outport  InitialOutput=0  VectorParamsAs1DForOutWhenUnconnected=off
  wires:
  Discrete Transfer Fcn/1 -> Out/1
  In/1 -> Discrete Transfer Fcn/1

== matlab function MODELSIMTOANHETHONG/Bộ tính từ thông,góc theta/MATLAB Function4 ==
  data: u input; y output
function y = fcn(u)
    if u<=0 
        y=u+2*pi;
    elseif u>=2*pi
            y = u-2*pi;
    else
y = u;
    end


end
